simulink model "project1_week3_part2"  (R2023b)
settings: Solver=VariableStepAuto  StartTime=0.0  StopTime=10.0  RelTol=1e-3
values from neighbouring files (symbols this model uses):
  A = [0.0, 100,0,100]    [P1_week3_code.m]
  b = [10,0.1]    [P1_week3_code.m]
  freq = [0.1,100]    [P1_week3_code.m]
  J = [100,0.01]    [P1_week3_code.m]
  w_0 = [10.0,0.0]    [P1_week3_code.m]
undefined symbols (not defined in the file or in its folder): control
settings Model: Creator=rahma  LastModifiedBy=rahma

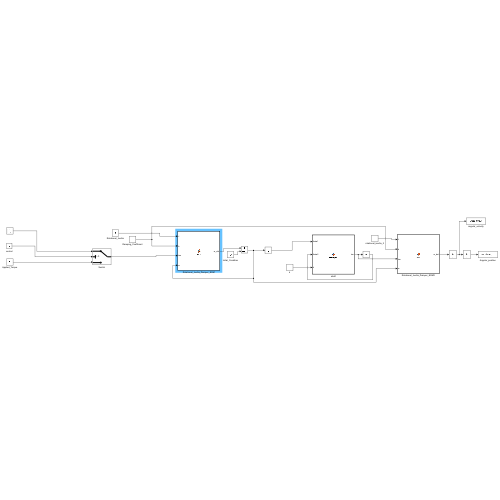
[thumbnail: Simulink's stored preview of the top-level diagram]
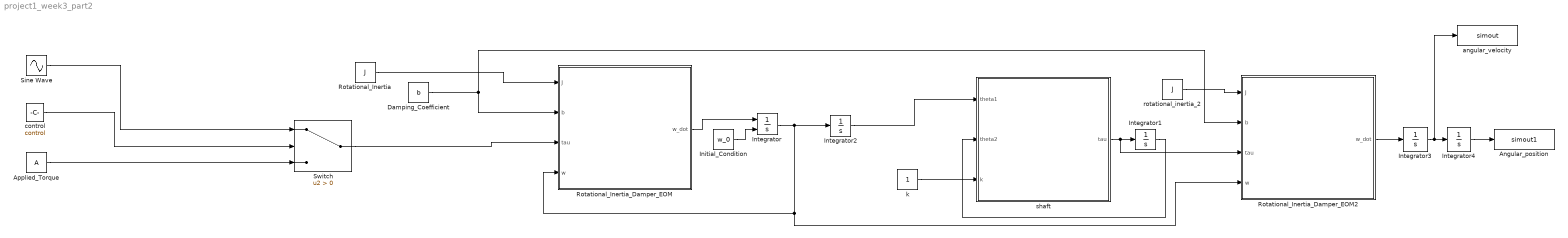
== system project1_week3_part2 ==
  Angular_position : ToWorkspace  VariableName=simout1  SaveFormat=Timeseries  SampleTime=-1
  Applied_Torque : Constant  Value=A
  Damping_Coefficient : Constant  Value=b
  Initial_Condition : Constant  Value=w_0
  Integrator : Integrator  InitialConditionSource=external
  Integrator{1..4} (4 alike) : Integrator
  Rotational_Inertia : Constant  Value=J
  Rotational_Inertia_Damper_EOM : MATLAB Function  TreatAsAtomicUnit=on
  Rotational_Inertia_Damper_EOM2 : MATLAB Function  TreatAsAtomicUnit=on
  Sine Wave : Sin  Amplitude=A  Frequency=freq  SampleTime=0
  Switch : Switch  Criteria=u2 > Threshold  SaturateOnIntegerOverflow=off  InputSameDT=off
  angular_velocity : ToWorkspace  VariableName=simout  SaveFormat=Timeseries  SampleTime=-1
  control : Constant  Value=control
  k : Constant
  rotational_inertia_2 : Constant  Value=J
  shaft : MATLAB Function  TreatAsAtomicUnit=on
  wires:
  Sine Wave/1 -> Switch/1
  Switch/1 -> Rotational_Inertia_Damper_EOM/3(tau)
  control/1 -> Switch/2
  Damping_Coefficient/1 -> Rotational_Inertia_Damper_EOM/2(b), Rotational_Inertia_Damper_EOM2/2(b)
  Integrator/1 -> Integrator2/1, Rotational_Inertia_Damper_EOM2/4(w), Rotational_Inertia_Damper_EOM/4(w)
  Rotational_Inertia/1 -> Rotational_Inertia_Damper_EOM/1(J)
  Applied_Torque/1 -> Switch/3
  Rotational_Inertia_Damper_EOM/1(w_dot) -> Integrator/1
  Initial_Condition/1 -> Integrator/2
  shaft/1(tau) -> Rotational_Inertia_Damper_EOM2/3(tau), Integrator1/1
  Integrator1/1 -> shaft/2(theta2)
  Integrator2/1 -> shaft/1(theta1)
  k/1 -> shaft/3(k)
  rotational_inertia_2/1 -> Rotational_Inertia_Damper_EOM2/1(J)
  Rotational_Inertia_Damper_EOM2/1(w_dot) -> Integrator3/1
  Integrator3/1 -> angular_velocity/1, Integrator4/1
  Integrator4/1 -> Angular_position/1

== matlab function project1_week3_part2/Rotational_Inertia_Damper_EOM2 ==
  data: J input; w_dot output; b input; tau input; w input
function w_dot = eom(J, b, tau, w)
% Recall EOM: J*w_dot = tau_applied - tau_damped
tau_damped = b.*w;
% tau = A.*sin(freq.*t);
w_dot = (1/J)*(tau - tau_damped);
end

== matlab function project1_week3_part2/Rotational_Inertia_Damper_EOM ==
  data: J input; w_dot output; b input; tau input; w input
function w_dot = eom(J, b, tau, w)
% Recall EOM: J*w_dot = tau_applied - tau_damped
tau_damped = b.*w;
% tau = A.*sin(freq.*t);
w_dot = (1/J)*(tau - tau_damped);
end

== matlab function project1_week3_part2/shaft ==
  data: theta1 input; tau output; theta2 input; k input
function tau = stiffness(theta1,theta2,k)
% Recall EOM: J*w_dot = tau_applied - tau_damped
tau=k*(theta1-theta2);
% tau = A.*sin(freq.*t);
end
